simulink model "sawtooth"  (R2015b)
settings: Solver=FixedStepAuto  StartTime=0.0  StopTime=500.0  RelTol=1e-3
libraries: fuzblock x1
settings Model: Creator=metalhead  LastModifiedBy=metalhead

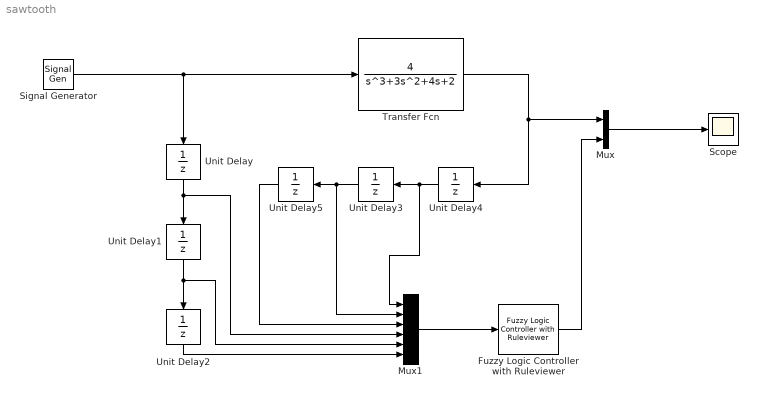
== system sawtooth ==
  Fuzzy Logic Controller with Ruleviewer : fuzblock/Fuzzy Logic  Controller  with Ruleviewer  fismatrix=fuzzymodel  Ts=1
  Mux : Mux  Inputs=2
  Mux1 : Mux  Inputs=6
  Scope : Scope
  Signal Generator : SignalGenerator  WaveForm=sawtooth  Units=rad/sec
  Transfer Fcn : TransferFcn  Numerator=[4]  Denominator=[1 3 4 2]
  Unit Delay{,1..5} (6 alike) : UnitDelay  SampleTime=-1
  wires:
  Signal Generator/1 -> Transfer Fcn/1, Unit Delay/1
  Unit Delay/1 -> Mux1/4, Unit Delay1/1
  Unit Delay1/1 -> Mux1/5, Unit Delay2/1
  Transfer Fcn/1 -> Mux/1, Unit Delay4/1
  Unit Delay4/1 -> Mux1/1, Unit Delay3/1
  Unit Delay3/1 -> Mux1/2, Unit Delay5/1
  Unit Delay5/1 -> Mux1/3
  Unit Delay2/1 -> Mux1/6
  Mux1/1 -> Fuzzy Logic Controller with Ruleviewer/1
  Fuzzy Logic Controller with Ruleviewer/1 -> Mux/2
  Mux/1 -> Scope/1
